simulink model "titled7"  (R2015b)
settings: Solver=FixedStepAuto  StartTime=0.0  StopTime=10.0  FixedStep=1/8000  RelTol=1e-3
libraries: dsparch4 x1, dspsrcs4 x1
settings Model: Creator=Lukas  LastModifiedBy=Lukas

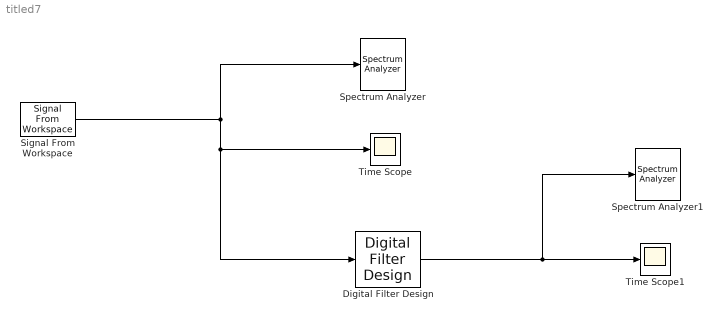
== system titled7 ==
  Digital Filter Design : dsparch4/Digital Filter Design  mwdsp_browser_bugfix_var=off
  Signal From Workspace : dspsrcs4/Signal From Workspace  X=signal6  Ts=1/8000  nsamps=1  OutputAfterFinalValue=Cyclic repetition  ignoreOrWarnInputAndFrameLengths=off  OutputFrames=off
  Spectrum Analyzer : SpectrumAnalyzer
  Spectrum Analyzer1 : SpectrumAnalyzer
  Time Scope : Scope
  Time Scope1 : Scope
  wires:
  Signal From Workspace/1 -> Spectrum Analyzer/1, Digital Filter Design/1, Time Scope/1
  Digital Filter Design/1 -> Spectrum Analyzer1/1, Time Scope1/1
